simulink model "ImpedanceControl"  (R2017a)
settings: Solver=ode23t  StartTime=0.0  StopTime=10.0  RelTol=1e-1
values from neighbouring files (symbols this model uses):
  Kd = 500*eye(6)    [Initial.m]
  Kp = 2500*eye(6)    [Initial.m]
  Md = 100*eye(6)    [Initial.m]
  Md_inv = inv(Md)    [Initial.m]
libraries: mblibv1 x72
(part 1 of 14)
settings Model: Creator=nathaliemajcherczyk  LastModifiedBy=Nathalie M
settings SolverCC: MaxConsecutiveMinStep=10

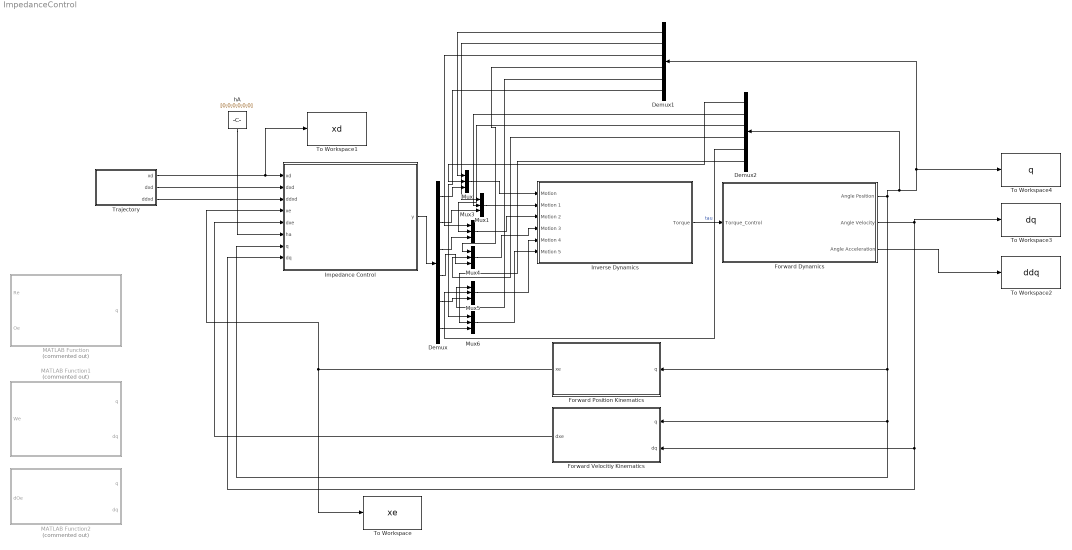
== system ImpedanceControl ==
  Demux : Demux  Outputs=6
  Demux1 : Demux  Outputs=6
  Demux2 : Demux  Outputs=6
  "Forward Dynamics " : Subsystem
  Forward Position Kinematics : MATLAB Function  TreatAsAtomicUnit=on
  Forward Velocitiy Kinematics : MATLAB Function  TreatAsAtomicUnit=on
  Impedance Control : Subsystem
  "Inverse Dynamics " : Subsystem
  MATLAB Function : MATLAB Function  Commented=on  TreatAsAtomicUnit=on
  MATLAB Function1 : MATLAB Function  Commented=on  TreatAsAtomicUnit=on
  MATLAB Function2 : MATLAB Function  Commented=on  TreatAsAtomicUnit=on
  Mux{,1,3..6} (6 alike) : Mux  Inputs=3
  To Workspace : ToWorkspace  VariableName=xe  SaveFormat=Timeseries  SampleTime=-1
  To Workspace1 : ToWorkspace  VariableName=xd  SaveFormat=Timeseries  SampleTime=-1
  To Workspace2 : ToWorkspace  VariableName=ddq  SaveFormat=Timeseries  SampleTime=-1
  To Workspace3 : ToWorkspace  VariableName=dq  SaveFormat=Timeseries  SampleTime=-1
  To Workspace4 : ToWorkspace  VariableName=q  SaveFormat=Timeseries  SampleTime=-1
  Trajectory : Subsystem
  hA : Constant  Value=[0;0;0;0;0;0]
  wires:
  "Forward Dynamics "/1("Angle Position ") -> Demux2/1, To Workspace4/1, Demux1/1, Forward Position Kinematics/1(q), Impedance Control/7(q), Forward Velocitiy Kinematics/1(q)
  "Forward Dynamics "/3(Angle Acceleration) -> To Workspace2/1
  "Forward Dynamics "/2(Angle Velocity) -> To Workspace3/1, Impedance Control/8(dq), Forward Velocitiy Kinematics/2(dq)
  "Inverse Dynamics "/1("Torque ") -> "Forward Dynamics "/1("Torque_Control ")  "tau"
  Impedance Control/1(y) -> Demux/1
  Forward Velocitiy Kinematics/1(dxe) -> Impedance Control/5(dxe)
  Forward Position Kinematics/1(xe) -> Impedance Control/4(xe), To Workspace/1
  hA/1 -> Impedance Control/6(ha)
  Trajectory/1(xd) -> To Workspace1/1, Impedance Control/1(xd)
  Trajectory/2(dxd) -> Impedance Control/2(dxd)
  Trajectory/3(ddxd) -> Impedance Control/3(ddxd)
  Demux/1 -> Mux/3
  Mux/1 -> "Inverse Dynamics "/1("Motion ")
  Demux1/1 -> Mux/1
  Demux2/1 -> Mux/2
  Demux/2 -> Mux1/3
  Mux1/1 -> "Inverse Dynamics "/2(Motion 1)
  Demux1/2 -> Mux1/1
  Demux2/2 -> Mux1/2
  Demux/3 -> Mux3/3
  Demux1/3 -> Mux3/1
  Demux2/3 -> Mux3/2
  Mux3/1 -> "Inverse Dynamics "/3(Motion 2)
  Demux/4 -> Mux4/3
  Mux4/1 -> "Inverse Dynamics "/4(Motion 3)
  Demux1/4 -> Mux4/1
  Demux2/4 -> Mux4/2
  Demux1/6 -> Mux6/1
  Demux/5 -> Mux5/3
  Mux5/1 -> "Inverse Dynamics "/5(Motion 4)
  Demux/6 -> Mux6/3
  Mux6/1 -> "Inverse Dynamics "/6(Motion 5)
  Demux2/6 -> Mux6/2
  Demux1/5 -> Mux5/1
  Demux2/5 -> Mux5/2

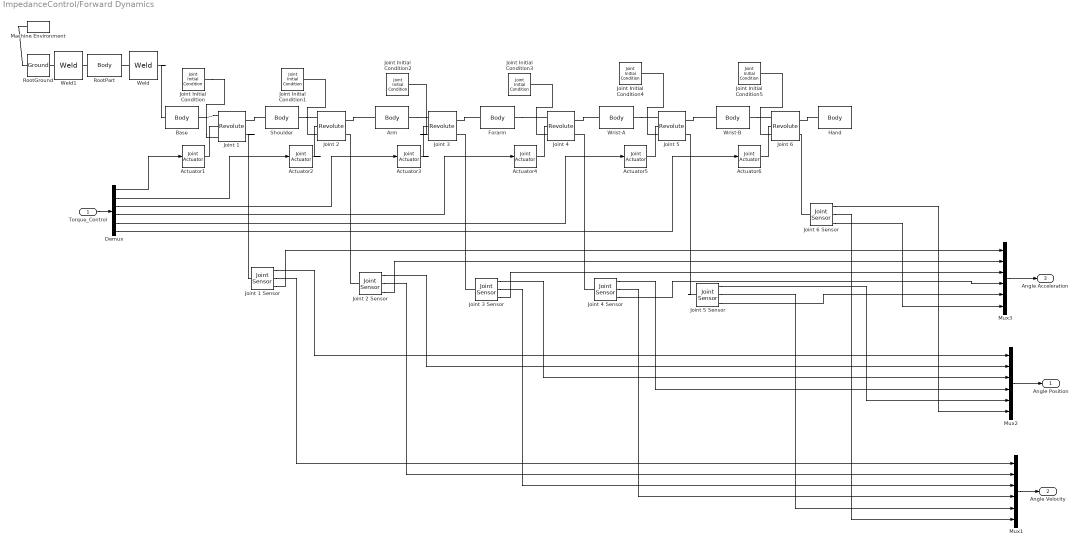
== system ImpedanceControl/Forward Dynamics  ==
  "Torque_Control " : Inport
  Actuator{1..6} (6 alike) : mblibv1/Sensors &  Actuators/Joint Actuator  UpdateFromCAD=off  PhysicalDomain=Mechanical  PortType=blob  ActuationStyle=Force  AngleUnits=deg  ArcVelocityUnits=deg/s  ArcAccelerationUnits=deg/s^2  CoordPositionUnits=m  VelocityUnits=m/s  AccelerationUnits=m/s^2  ForceUnits=N  TorqueUnits=N-m  ActiveIO=on  Width=1  DialogClass=MechanicalActuatorBlock  Primitive=R1  ReferenceFrame=Absolute (World)
      settings: SourceProductName=Simscape Multibody  SourceProductBaseCode=MS
  Arm : mblibv1/Bodies/Body  LConnTagsString=CS2  RConnTagsString=CS3  UpdateFromCAD=on  DialogClass=MechanicalBodyBlock  Mass=1.056  MassUnits=kg  InertiaUnits=kg*m^2  Inertia=[0.0375645,-1.33324e-07,0.000108785;-1.33324e-07,0.0372402,-2.39225e-07;0.000108785,-2.39225e-07,0.00059301]  Shape=Cylinder  ShapeDims=[1 1]  ShapeUnits=m  ShapeUse=false  Density=1  DensityUnits=kg/m^3  DensityUse=false  GraphicsMode=GFXFILE  GraphicsFileName=Jaco_3_7 - arm_ass-1.STL  BodyColorSelMode=COLORPALETTE  BodyColor=[0.752941;0.752941;0.752941]  AttachedToCS=CS1  CG=Right$CG$[0.10282 0.0944444 0.508793]$WORLD$WORLD$m$[0.695251 0.715707 -0.0662524;0.718767 -0.692291 0.0640847;0 -0.092175 -0.995743]$3x3 Transform$rad$WORLD$false$none  WorkingFrames=Right$CS1$[-0.183907 0.105598 0.903425]$WORLD$WORLD$m$[0.695251 0.715707 -0.0662524;0.718767 -0.692291 0.0640847;0 -0.092175 -0.995743]$3x3 Transform$rad$WORLD$false$none#Left$CS2$[0.0767642 0.095252 0.300589]$WORLD$WORLD$m$[1 0 0;0 1 0;0 0 1]$3x3 Transform$rad$WORLD$true$none#Right$CS3$[0.10358 0.0686179 0.708843]$WORLD$WORLD$m$[1 0 0;0 1 0;0 0 1]$3x3 Transform$rad$WORLD$true$none  CGPos=[0.10282 0.0944444 0.508793]  CGRot=[0.695251 0.715707 -0.0662524;0.718767 -0.692291 0.0640847;0 -0.092175 -0.995743]  CS0Pos=[]  CS0Rot=[]  CS1Pos=[-0.183907 0.105598 0.903425]  CS1Rot=[0.695251 0.715707 -0.0662524;0.718767 -0.692291 0.0640847;0 -0.092175 -0.995743]  CS2Pos=[0.0767642 0.095252 0.300589]  CS2Rot=[1 0 0;0 1 0;0 0 1]  CS3Pos=[0.10358 0.0686179 0.708843]  CS3Rot=[1 0 0;0 1 0;0 0 1]  CS4Pos=[]  CS4Rot=[]  CS5Pos=[]  CS5Rot=[]  CS6Pos=[]  CS6Rot=[]  CS7Pos=[]  CS7Rot=[]  CS8Pos=[]  CS8Rot=[]  CS9Pos=[]  CS9Rot=[]  CS10Pos=[]  CS10Rot=[]  CS11Pos=[]  CS11Rot=[]  CS12Pos=[]  CS12Rot=[]  CS13Pos=[]  CS13Rot=[]  CS14Pos=[]  CS14Rot=[]  CS15Pos=[]  CS15Rot=[]  CS16Pos=[]  CS16Rot=[]  CS17Pos=[]  CS17Rot=[]  CS18Pos=[]  CS18Rot=[]  CS19Pos=[]  CS19Rot=[]  CS20Pos=[]  CS20Rot=[]
      settings: SourceProductName=Simscape Multibody  SourceProductBaseCode=MS
  Base : mblibv1/Bodies/Body  LConnTagsString=CS2  RConnTagsString=CS3  UpdateFromCAD=on  DialogClass=MechanicalBodyBlock  Mass=0.570939  MassUnits=kg  InertiaUnits=kg*m^2  Inertia=[0.00175947,1.92772e-07,-3.1782e-05;1.92772e-07,0.00176256,-3.18122e-05;-3.1782e-05,-3.18122e-05,0.000478232]  Shape=Cylinder  ShapeDims=[1 1]  ShapeUnits=m  ShapeUse=false  Density=1  DensityUnits=kg/m^3  DensityUse=false  GraphicsMode=GFXFILE  GraphicsFileName=Jaco_3_7 - base_ass-1.STL  BodyColorSelMode=COLORPALETTE  BodyColor=[0.752941;0.752941;0.752941]  AttachedToCS=CS1  CG=Right$CG$[0.0747134 0.093124 0.128067]$WORLD$WORLD$m$[1 0 0;0 1 0;0 0 1]$3x3 Transform$rad$WORLD$false$none  WorkingFrames=Right$CS1$[0.106448 0.0299726 -0.0762042]$WORLD$WORLD$m$[1 0 0;0 1 0;0 0 1]$3x3 Transform$rad$WORLD$false$none#Left$CS2$[0.0747134 0.093124 0.128067]$WORLD$WORLD$m$[1 0 0;0 1 0;0 0 1]$3x3 Transform$rad$WORLD$true$none#Right$CS3$[0.0753736 0.0938145 0.182089]$WORLD$WORLD$m$[1 0 0;0 1 0;0 0 1]$3x3 Transform$rad$WORLD$true$none  CGPos=[0.0747134 0.093124 0.128067]  CGRot=[1 0 0;0 1 0;0 0 1]  CS0Pos=[]  CS0Rot=[]  CS1Pos=[0.106448 0.0299726 -0.0762042]  CS1Rot=[1 0 0;0 1 0;0 0 1]  CS2Pos=[0.0747134 0.093124 0.128067]  CS2Rot=[1 0 0;0 1 0;0 0 1]  CS3Pos=[0.0753736 0.0938145 0.182089]  CS3Rot=[1 0 0;0 1 0;0 0 1]  CS4Pos=[]  CS4Rot=[]  CS5Pos=[]  CS5Rot=[]  CS6Pos=[]  CS6Rot=[]  CS7Pos=[]  CS7Rot=[]  CS8Pos=[]  CS8Rot=[]  CS9Pos=[]  CS9Rot=[]  CS10Pos=[]  CS10Rot=[]  CS11Pos=[]  CS11Rot=[]  CS12Pos=[]  CS12Rot=[]  CS13Pos=[]  CS13Rot=[]  CS14Pos=[]  CS14Rot=[]  CS15Pos=[]  CS15Rot=[]  CS16Pos=[]  CS16Rot=[]  CS17Pos=[]  CS17Rot=[]  CS18Pos=[]  CS18Rot=[]  CS19Pos=[]  CS19Rot=[]  CS20Pos=[]  CS20Rot=[]
      settings: SourceProductName=Simscape Multibody  SourceProductBaseCode=MS
  Demux : Demux  Outputs=6
  Forarm : mblibv1/Bodies/Body  LConnTagsString=CS2  RConnTagsString=CS3  UpdateFromCAD=on  DialogClass=MechanicalBodyBlock  Mass=0.735414  MassUnits=kg  InertiaUnits=kg*m^2  Inertia=[0.00626271,-0.000115651,1.81814e-08;-0.000115651,0.000377159,4.13244e-07;1.81814e-08,4.13244e-07,0.00610747]  Shape=Cylinder  ShapeDims=[1 1]  ShapeUnits=m  ShapeUse=false  Density=1  DensityUnits=kg/m^3  DensityUse=false  GraphicsMode=GFXFILE  GraphicsFileName=Jaco_3_7 - forarm_ass-1.STL  BodyColorSelMode=COLORPALETTE  BodyColor=[0.752941;0.752941;0.752941]  AttachedToCS=CS1  CG=Right$CG$[0.142291 0.0111153 0.740623]$WORLD$WORLD$m$[0.695251 0.650811 0.305076;0.718767 -0.629518 -0.295094;0 0.424443 -0.905455]$3x3 Transform$rad$WORLD$false$none  WorkingFrames=Right$CS1$[-0.0310579 0.0970807 0.899014]$WORLD$WORLD$m$[0.695251 0.650811 0.305076;0.718767 -0.629518 -0.295094;0 0.424443 -0.905455]$3x3 Transform$rad$WORLD$false$none#Left$CS2$[0.10358 0.0686179 0.708843]$WORLD$WORLD$m$[1 0 0;0 1 0;0 0 1]$3x3 Transform$rad$WORLD$true$none#Right$CS3$[0.230802 -0.0700932 0.796915]$WORLD$WORLD$m$[1 0 0;0 1 0;0 0 1]$3x3 Transform$rad$WORLD$true$none  CGPos=[0.142291 0.0111153 0.740623]  CGRot=[0.695251 0.650811 0.305076;0.718767 -0.629518 -0.295094;0 0.424443 -0.905455]  CS0Pos=[]  CS0Rot=[]  CS1Pos=[-0.0310579 0.0970807 0.899014]  CS1Rot=[0.695251 0.650811 0.305076;0.718767 -0.629518 -0.295094;0 0.424443 -0.905455]  CS2Pos=[0.10358 0.0686179 0.708843]  CS2Rot=[1 0 0;0 1 0;0 0 1]  CS3Pos=[0.230802 -0.0700932 0.796915]  CS3Rot=[1 0 0;0 1 0;0 0 1]  CS4Pos=[]  CS4Rot=[]  CS5Pos=[]  CS5Rot=[]  CS6Pos=[]  CS6Rot=[]  CS7Pos=[]  CS7Rot=[]  CS8Pos=[]  CS8Rot=[]  CS9Pos=[]  CS9Rot=[]  CS10Pos=[]  CS10Rot=[]  CS11Pos=[]  CS11Rot=[]  CS12Pos=[]  CS12Rot=[]  CS13Pos=[]  CS13Rot=[]  CS14Pos=[]  CS14Rot=[]  CS15Pos=[]  CS15Rot=[]  CS16Pos=[]  CS16Rot=[]  CS17Pos=[]  CS17Rot=[]  CS18Pos=[]  CS18Rot=[]  CS19Pos=[]  CS19Rot=[]  CS20Pos=[]  CS20Rot=[]
      settings: SourceProductName=Simscape Multibody  SourceProductBaseCode=MS
  Hand : mblibv1/Bodies/Body  LConnTagsString=CS2  UpdateFromCAD=on  DialogClass=MechanicalBodyBlock  Mass=0.395999  MassUnits=kg  InertiaUnits=kg*m^2  Inertia=[0.00124769,-0.000197969,-5.51354e-06;-0.000197969,0.000409818,-2.12169e-05;-5.51354e-06,-2.12169e-05,0.00139509]  Shape=Cylinder  ShapeDims=[1 1]  ShapeUnits=m  ShapeUse=false  Density=1  DensityUnits=kg/m^3  DensityUse=false  GraphicsMode=GFXFILE  GraphicsFileName=Jaco_3_7 - Hand_ass-1.STL  BodyColorSelMode=COLORPALETTE  BodyColor=[0.752941;0.752941;0.752941]  AttachedToCS=CS1  CG=Right$CG$[0.35442 -0.232757 0.799495]$WORLD$WORLD$m$[-0.439555 0.858973 -0.262597;-0.828489 -0.500657 -0.250895;-0.346983 0.107276 0.931716]$3x3 Transform$rad$WORLD$false$none  WorkingFrames=Right$CS1$[0.362295 -0.115327 0.65151]$WORLD$WORLD$m$[-0.439555 0.858973 -0.262597;-0.828489 -0.500657 -0.250895;-0.346983 0.107276 0.931716]$3x3 Transform$rad$WORLD$false$none#Left$CS2$[0.306767 -0.196631 0.795235]$WORLD$WORLD$m$[1 0 0;0 1 0;0 0 1]$3x3 Transform$rad$WORLD$true$none  CGPos=[0.35442 -0.232757 0.799495]  CGRot=[-0.439555 0.858973 -0.262597;-0.828489 -0.500657 -0.250895;-0.346983 0.107276 0.931716]  CS0Pos=[]  CS0Rot=[]  CS1Pos=[0.362295 -0.115327 0.65151]  CS1Rot=[-0.439555 0.858973 -0.262597;-0.828489 -0.500657 -0.250895;-0.346983 0.107276 0.931716]  CS2Pos=[0.306767 -0.196631 0.795235]  CS2Rot=[1 0 0;0 1 0;0 0 1]  CS3Pos=[]  CS3Rot=[]  CS4Pos=[]  CS4Rot=[]  CS5Pos=[]  CS5Rot=[]  CS6Pos=[]  CS6Rot=[]  CS7Pos=[]  CS7Rot=[]  CS8Pos=[]  CS8Rot=[]  CS9Pos=[]  CS9Rot=[]  CS10Pos=[]  CS10Rot=[]  CS11Pos=[]  CS11Rot=[]  CS12Pos=[]  CS12Rot=[]  CS13Pos=[]  CS13Rot=[]  CS14Pos=[]  CS14Rot=[]  CS15Pos=[]  CS15Rot=[]  CS16Pos=[]  CS16Rot=[]  CS17Pos=[]  CS17Rot=[]  CS18Pos=[]  CS18Rot=[]  CS19Pos=[]  CS19Rot=[]  CS20Pos=[]  CS20Rot=[]
      settings: SourceProductName=Simscape Multibody  SourceProductBaseCode=MS
  Joint 1 : mblibv1/Joints/Revolute  LConnTagsString=__newl0|SA1|SA2  RConnTagsString=__newr0|SA1  UpdateFromCAD=on  NumSAPorts=3  CutJoint=off  MarkAsCut=off  Primitives=prismatic  PrimitiveProps=R1$World$[0,0,1]$revolute  DialogClass=JointBlock  R1Axis=[0,0,1]
      settings: SourceProductName=Simscape Multibody  SourceProductBaseCode=MS
  Joint 1 Sensor : mblibv1/Sensors &  Actuators/Joint Sensor  UpdateFromCAD=off  PhysicalDomain=Mechanical  PortType=blob  Muxed=off  Pose=off  Angle=on  AngleUnits=deg  ArcVelocity=on  ArcVelocityUnits=deg/s  ArcAcceleration=on  ArcAccelerationUnits=deg/s^2  CoordPosition=on  CoordPositionUnits=m  Velocity=off  VelocityUnits=m/s  Acceleration=off  AccelerationUnits=m/s^2  Quaternion=on  QuaternionDT=off  QuaternionDDT=off  QuaternionUnits=off  OutputVector=[1]  ActiveIO=on  Width=3  DialogClass=MechanicalSensorBlock  Primitive=R1  Force=off  ForceUnits=N  Torque=off  TorqueUnits=N*m  ReferenceFrame=Absolute (World)  ReactionSensedSide=Base  ReactionReferenceFrame=Absolute (World)  ReactionForce=off  ReactionForceUnits=N  ReactionMoment=off  ReactionMomentUnits=N*m
      settings: SourceProductName=Simscape Multibody  SourceProductBaseCode=MS
  Joint 2 : mblibv1/Joints/Revolute  LConnTagsString=__newl0|SA1|SA2  RConnTagsString=__newr0|SA1  UpdateFromCAD=on  NumSAPorts=3  CutJoint=off  MarkAsCut=off  Primitives=prismatic  PrimitiveProps=R1$World$[0.695251,0.718767,0]$revolute  DialogClass=JointBlock  R1Axis=[0.695251,0.718767,0]
      settings: SourceProductName=Simscape Multibody  SourceProductBaseCode=MS
  Joint 2 Sensor : mblibv1/Sensors &  Actuators/Joint Sensor  UpdateFromCAD=off  PhysicalDomain=Mechanical  PortType=blob  Muxed=off  Pose=off  Angle=on  AngleUnits=deg  ArcVelocity=on  ArcVelocityUnits=deg/s  ArcAcceleration=on  ArcAccelerationUnits=deg/s^2  CoordPosition=on  CoordPositionUnits=m  Velocity=off  VelocityUnits=m/s  Acceleration=off  AccelerationUnits=m/s^2  Quaternion=on  QuaternionDT=off  QuaternionDDT=off  QuaternionUnits=off  OutputVector=[1]  ActiveIO=on  Width=3  DialogClass=MechanicalSensorBlock  Primitive=R1  Force=off  ForceUnits=N  Torque=off  TorqueUnits=N*m  ReferenceFrame=Absolute (World)  ReactionSensedSide=Base  ReactionReferenceFrame=Absolute (World)  ReactionForce=off  ReactionForceUnits=N  ReactionMoment=off  ReactionMomentUnits=N*m
      settings: SourceProductName=Simscape Multibody  SourceProductBaseCode=MS
  Joint 3 : mblibv1/Joints/Revolute  LConnTagsString=__newl0|SA1|SA2  RConnTagsString=__newr0|SA1  UpdateFromCAD=on  NumSAPorts=3  CutJoint=off  MarkAsCut=off  Primitives=prismatic  PrimitiveProps=R1$World$[-0.695251,-0.718767,0]$revolute  DialogClass=JointBlock  R1Axis=[-0.695251,-0.718767,0]
      settings: SourceProductName=Simscape Multibody  SourceProductBaseCode=MS
  Joint 3 Sensor : mblibv1/Sensors &  Actuators/Joint Sensor  UpdateFromCAD=off  PhysicalDomain=Mechanical  PortType=blob  Muxed=off  Pose=off  Angle=on  AngleUnits=deg  ArcVelocity=on  ArcVelocityUnits=deg/s  ArcAcceleration=on  ArcAccelerationUnits=deg/s^2  CoordPosition=on  CoordPositionUnits=m  Velocity=off  VelocityUnits=m/s  Acceleration=off  AccelerationUnits=m/s^2  Quaternion=on  QuaternionDT=off  QuaternionDDT=off  QuaternionUnits=off  OutputVector=[1]  ActiveIO=on  Width=3  DialogClass=MechanicalSensorBlock  Primitive=R1  Force=off  ForceUnits=N  Torque=off  TorqueUnits=N*m  ReferenceFrame=Absolute (World)  ReactionSensedSide=Base  ReactionReferenceFrame=Absolute (World)  ReactionForce=off  ReactionForceUnits=N  ReactionMoment=off  ReactionMomentUnits=N*m
      settings: SourceProductName=Simscape Multibody  SourceProductBaseCode=MS
  Joint 4 : mblibv1/Joints/Revolute  LConnTagsString=__newl0|SA1|SA2  RConnTagsString=__newr0|SA1  UpdateFromCAD=on  NumSAPorts=3  CutJoint=off  MarkAsCut=off  Primitives=prismatic  PrimitiveProps=R1$World$[0.650811,-0.629518,0.424443]$revolute  DialogClass=JointBlock  R1Axis=[0.650811,-0.629518,0.424443]
      settings: SourceProductName=Simscape Multibody  SourceProductBaseCode=MS
  Joint 4 Sensor : mblibv1/Sensors &  Actuators/Joint Sensor  UpdateFromCAD=off  PhysicalDomain=Mechanical  PortType=blob  Muxed=off  Pose=off  Angle=on  AngleUnits=deg  ArcVelocity=on  ArcVelocityUnits=deg/s  ArcAcceleration=on  ArcAccelerationUnits=deg/s^2  CoordPosition=on  CoordPositionUnits=m  Velocity=off  VelocityUnits=m/s  Acceleration=off  AccelerationUnits=m/s^2  Quaternion=on  QuaternionDT=off  QuaternionDDT=off  QuaternionUnits=off  OutputVector=[1]  ActiveIO=on  Width=3  DialogClass=MechanicalSensorBlock  Primitive=R1  Force=off  ForceUnits=N  Torque=off  TorqueUnits=N*m  ReferenceFrame=Absolute (World)  ReactionSensedSide=Base  ReactionReferenceFrame=Absolute (World)  ReactionForce=off  ReactionForceUnits=N  ReactionMoment=off  ReactionMomentUnits=N*m
      settings: SourceProductName=Simscape Multibody  SourceProductBaseCode=MS
  Joint 5 : mblibv1/Joints/Revolute  LConnTagsString=__newl0|SA1|SA2  RConnTagsString=__newr0|SA1  UpdateFromCAD=on  NumSAPorts=3  CutJoint=off  MarkAsCut=off  Primitives=prismatic  PrimitiveProps=R1$World$[0.15169,-0.946456,-0.284976]$revolute  DialogClass=JointBlock  R1Axis=[0.15169,-0.946456,-0.284976]
      settings: SourceProductName=Simscape Multibody  SourceProductBaseCode=MS
  Joint 5 Sensor : mblibv1/Sensors &  Actuators/Joint Sensor  UpdateFromCAD=off  PhysicalDomain=Mechanical  PortType=blob  Muxed=off  Pose=off  Angle=on  AngleUnits=deg  ArcVelocity=on  ArcVelocityUnits=deg/s  ArcAcceleration=on  ArcAccelerationUnits=deg/s^2  CoordPosition=on  CoordPositionUnits=m  Velocity=off  VelocityUnits=m/s  Acceleration=off  AccelerationUnits=m/s^2  Quaternion=on  QuaternionDT=off  QuaternionDDT=off  QuaternionUnits=off  OutputVector=[1]  ActiveIO=on  Width=3  DialogClass=MechanicalSensorBlock  Primitive=R1  Force=off  ForceUnits=N  Torque=off  TorqueUnits=N*m  ReferenceFrame=Absolute (World)  ReactionSensedSide=Base  ReactionReferenceFrame=Absolute (World)  ReactionForce=off  ReactionForceUnits=N  ReactionMoment=off  ReactionMomentUnits=N*m
      settings: SourceProductName=Simscape Multibody  SourceProductBaseCode=MS
  Joint 6 : mblibv1/Joints/Revolute  LConnTagsString=__newl0|SA1|SA2  RConnTagsString=__newr0|SA1  UpdateFromCAD=on  NumSAPorts=3  CutJoint=off  MarkAsCut=off  Primitives=prismatic  PrimitiveProps=R1$World$[0.858973,-0.500657,0.107276]$revolute  DialogClass=JointBlock  R1Axis=[0.858973,-0.500657,0.107276]
      settings: SourceProductName=Simscape Multibody  SourceProductBaseCode=MS
  Joint 6 Sensor : mblibv1/Sensors &  Actuators/Joint Sensor  UpdateFromCAD=off  PhysicalDomain=Mechanical  PortType=blob  Muxed=off  Pose=off  Angle=on  AngleUnits=deg  ArcVelocity=on  ArcVelocityUnits=deg/s  ArcAcceleration=on  ArcAccelerationUnits=deg/s^2  CoordPosition=on  CoordPositionUnits=m  Velocity=off  VelocityUnits=m/s  Acceleration=off  AccelerationUnits=m/s^2  Quaternion=on  QuaternionDT=off  QuaternionDDT=off  QuaternionUnits=off  OutputVector=[1]  ActiveIO=on  Width=3  DialogClass=MechanicalSensorBlock  Primitive=R1  Force=off  ForceUnits=N  Torque=off  TorqueUnits=N*m  ReferenceFrame=Absolute (World)  ReactionSensedSide=Base  ReactionReferenceFrame=Absolute (World)  ReactionForce=off  ReactionForceUnits=N  ReactionMoment=off  ReactionMomentUnits=N*m
      settings: SourceProductName=Simscape Multibody  SourceProductBaseCode=MS
  Joint Initial Condition : mblibv1/Sensors &  Actuators/Joint Initial Condition  UpdateFromCAD=off  LeftPortType=blob  RightPortType=blob  PhysicalDomain=mechanical  DialogClass=InitialConditionBlock  InitialConditions=P1$false$0$m$deg$0$m/s$deg/s#P2$false$0$m$deg$0$m/s$deg/s#P3$false$0$m$deg$0$m/s$deg/s#R1$true$0.81$m$rad$0$m/s$rad/s#R2$false$0$m$deg$0$m/s$deg/s#R3$false$0$m$deg$0$m/s$deg/s#S$false$0$m$deg$0$m/s$deg/s  P1PIC=0  P1VIC=0  P2PIC=0  P2VIC=0  P3PIC=0  P3VIC=0  R1PIC=0.81  R1VIC=0  R2PIC=0  R2VIC=0  R3PIC=0  R3VIC=0  SPIC=0  SVIC=0
      settings: SourceProductName=Simscape Multibody  SourceProductBaseCode=MS
  Joint Initial Condition1 : mblibv1/Sensors &  Actuators/Joint Initial Condition  UpdateFromCAD=off  LeftPortType=blob  RightPortType=blob  PhysicalDomain=mechanical  DialogClass=InitialConditionBlock  InitialConditions=P1$false$0$m$deg$0$m/s$deg/s#P2$false$0$m$deg$0$m/s$deg/s#P3$false$0$m$deg$0$m/s$deg/s#R1$true$-0.6915$m$rad$0$m/s$rad/s#R2$false$0$m$deg$0$m/s$deg/s#R3$false$0$m$deg$0$m/s$deg/s#S$false$0$m$deg$0$m/s$deg/s  P1PIC=0  P1VIC=0  P2PIC=0  P2VIC=0  P3PIC=0  P3VIC=0  R1PIC=-0.6915  R1VIC=0  R2PIC=0  R2VIC=0  R3PIC=0  R3VIC=0  SPIC=0  SVIC=0
      settings: SourceProductName=Simscape Multibody  SourceProductBaseCode=MS
  Joint Initial Condition2 : mblibv1/Sensors &  Actuators/Joint Initial Condition  UpdateFromCAD=off  LeftPortType=blob  RightPortType=blob  PhysicalDomain=mechanical  DialogClass=InitialConditionBlock  InitialConditions=P1$false$0$m$deg$0$m/s$deg/s#P2$false$0$m$deg$0$m/s$deg/s#P3$false$0$m$deg$0$m/s$deg/s#R1$true$1.5708$m$rad$0.2$m/s$rad/s#R2$false$0$m$deg$0$m/s$deg/s#R3$false$0$m$deg$0$m/s$deg/s#S$false$0$m$deg$0$m/s$deg/s  P1PIC=0  P1VIC=0  P2PIC=0  P2VIC=0  P3PIC=0  P3VIC=0  R1PIC=1.5708  R1VIC=0.2  R2PIC=0  R2VIC=0  R3PIC=0  R3VIC=0  SPIC=0  SVIC=0
      settings: SourceProductName=Simscape Multibody  SourceProductBaseCode=MS
  Joint Initial Condition3 : mblibv1/Sensors &  Actuators/Joint Initial Condition  UpdateFromCAD=off  LeftPortType=blob  RightPortType=blob  PhysicalDomain=mechanical  DialogClass=InitialConditionBlock  InitialConditions=P1$false$0$m$deg$0$m/s$deg/s#P2$false$0$m$deg$0$m/s$deg/s#P3$false$0$m$deg$0$m/s$deg/s#R1$true$3.1415$m$rad$0$m/s$rad/s#R2$false$0$m$deg$0$m/s$deg/s#R3$false$0$m$deg$0$m/s$deg/s#S$false$0$m$deg$0$m/s$deg/s  P1PIC=0  P1VIC=0  P2PIC=0  P2VIC=0  P3PIC=0  P3VIC=0  R1PIC=3.1415  R1VIC=0  R2PIC=0  R2VIC=0  R3PIC=0  R3VIC=0  SPIC=0  SVIC=0
      settings: SourceProductName=Simscape Multibody  SourceProductBaseCode=MS
  Joint Initial Condition4 : mblibv1/Sensors &  Actuators/Joint Initial Condition  UpdateFromCAD=off  LeftPortType=blob  RightPortType=blob  PhysicalDomain=mechanical  DialogClass=InitialConditionBlock  InitialConditions=P1$false$0$m$deg$0$m/s$deg/s#P2$false$0$m$deg$0$m/s$deg/s#P3$false$0$m$deg$0$m/s$deg/s#R1$true$-1.70256$m$rad$0$m/s$deg/s#R2$false$0$m$deg$0$m/s$deg/s#R3$false$0$m$deg$0$m/s$deg/s#S$false$0$m$deg$0$m/s$deg/s  P1PIC=0  P1VIC=0  P2PIC=0  P2VIC=0  P3PIC=0  P3VIC=0  R1PIC=-1.70256  R1VIC=0  R2PIC=0  R2VIC=0  R3PIC=0  R3VIC=0  SPIC=0  SVIC=0
      settings: SourceProductName=Simscape Multibody  SourceProductBaseCode=MS
  Joint Initial Condition5 : mblibv1/Sensors &  Actuators/Joint Initial Condition  UpdateFromCAD=off  LeftPortType=blob  RightPortType=blob  PhysicalDomain=mechanical  DialogClass=InitialConditionBlock  InitialConditions=P1$false$0$m$deg$0$m/s$deg/s#P2$false$0$m$deg$0$m/s$deg/s#P3$false$0$m$deg$0$m/s$deg/s#R1$true$0.8222$m$rad$0$m/s$rad/s#R2$false$0$m$deg$0$m/s$deg/s#R3$false$0$m$deg$0$m/s$deg/s#S$false$0$m$deg$0$m/s$deg/s  P1PIC=0  P1VIC=0  P2PIC=0  P2VIC=0  P3PIC=0  P3VIC=0  R1PIC=0.8222  R1VIC=0  R2PIC=0  R2VIC=0  R3PIC=0  R3VIC=0  SPIC=0  SVIC=0
      settings: SourceProductName=Simscape Multibody  SourceProductBaseCode=MS
  Machine Environment : mblibv1/Bodies/Machine Environment  PortType=env  PhysicalDomain=Mechanical  DialogTemplateClass=MECH.MachineEnvironment  SyncWhenCopied=off  Gravity=[0 0 -9.81]  GravityUnits=m/s^2  GravityAsSignal=off  Dimensionality=Auto-detect  AnalysisType=Forward dynamics  LinearAssemblyTolerance=1e-3  LinearAssemblyToleranceUnits=m  AngularAssemblyTolerance=1e-3  AngularAssemblyToleranceUnits=rad  ConstraintSolverType=Stabilizing  ConstraintRelTolerance=1e-4  ConstraintAbsTolerance=1e-4  UseRobustSingularityHandling=off  RedundancyAnalysisToleranceType=Automatically select tolerance  RedundancyAnalysisTolerance=1e-14  StatePerturbationType=Fixed  PerturbationSize=1e-5  VisualizeMachine=on  BodyVisualizationType=Use model default body geometries  BodyColorSelMode=Use model default  DefaultBodyColor=[1 0 0]
      settings: SourceProductName=Simscape Multibody  SourceProductBaseCode=MS
  Mux1 : Mux  Inputs=6
  Mux2 : Mux  Inputs=6
  Mux3 : Mux  Inputs=6
  RootGround : mblibv1/Bodies/Ground  UpdateFromCAD=on  LeftPortType=env  RightPortType=workingframe  PhysicalDomain=Mechanical  DialogClass=GroundBlock  CoordPosition=[0.154743,0.00421299,0.535333]  CoordPositionUnits=m  StateVectorMgrId=0  MachineId=[1 0]  ShowEnvPort=on  ParameterChecksum=[3417922130, 2383928924, 3577010570, 1911939694]  TopologyChecksum=[2654763649, 4205204799, 1514762018, 2254763851]
      settings: SourceProductName=Simscape Multibody  SourceProductBaseCode=MS
  RootPart : mblibv1/Bodies/Body  LConnTagsString=CS3  RConnTagsString=CS2  UpdateFromCAD=on  DialogClass=MechanicalBodyBlock  Mass=0  MassUnits=kg  InertiaUnits=kg*m^2  Inertia=[0,0,0;0,0,0;0,0,0]  Shape=Cylinder  ShapeDims=[1 1]  ShapeUnits=m  ShapeUse=false  Density=1  DensityUnits=kg/m^3  DensityUse=false  GraphicsMode=MACHINE_DEFAULT  BodyColorSelMode=MACHINE_DEFAULT  BodyColor=[1;0;0]  AttachedToCS=CS1  CG=Right$CG$[0.154743 0.00421299 0.535333]$WORLD$WORLD$m$[1 0 0;0 1 0;0 0 1]$3x3 Transform$rad$WORLD$false$none  WorkingFrames=Right$CS1$[0 0 0]$WORLD$WORLD$m$[1 0 0;0 1 0;0 0 1]$3x3 Transform$rad$WORLD$false$none#Right$CS2$[0.0747134 0.093124 0.128067]$WORLD$WORLD$m$[1 0 0;0 1 0;0 0 1]$3x3 Transform$rad$WORLD$true$none#Left$CS3$[0.154743 0.00421299 0.535333]$WORLD$WORLD$m$[1 0 0;0 1 0;0 0 1]$3x3 Transform$rad$WORLD$true$none  CGPos=[0.154743 0.00421299 0.535333]  CGRot=[1 0 0;0 1 0;0 0 1]  CS0Pos=[]  CS0Rot=[]  CS1Pos=[0 0 0]  CS1Rot=[1 0 0;0 1 0;0 0 1]  CS2Pos=[0.0747134 0.093124 0.128067]  CS2Rot=[1 0 0;0 1 0;0 0 1]  CS3Pos=[0.154743 0.00421299 0.535333]  CS3Rot=[1 0 0;0 1 0;0 0 1]  CS4Pos=[]  CS4Rot=[]  CS5Pos=[]  CS5Rot=[]  CS6Pos=[]  CS6Rot=[]  CS7Pos=[]  CS7Rot=[]  CS8Pos=[]  CS8Rot=[]  CS9Pos=[]  CS9Rot=[]  CS10Pos=[]  CS10Rot=[]  CS11Pos=[]  CS11Rot=[]  CS12Pos=[]  CS12Rot=[]  CS13Pos=[]  CS13Rot=[]  CS14Pos=[]  CS14Rot=[]  CS15Pos=[]  CS15Rot=[]  CS16Pos=[]  CS16Rot=[]  CS17Pos=[]  CS17Rot=[]  CS18Pos=[]  CS18Rot=[]  CS19Pos=[]  CS19Rot=[]  CS20Pos=[]  CS20Rot=[]
      settings: SourceProductName=Simscape Multibody  SourceProductBaseCode=MS
  Shoulder : mblibv1/Bodies/Body  LConnTagsString=CS3  RConnTagsString=CS2  UpdateFromCAD=on  DialogClass=MechanicalBodyBlock  Mass=0.813994  MassUnits=kg  InertiaUnits=kg*m^2  Inertia=[0.0026546,0.000304923,5.38935e-08;0.000304923,0.000595598,-3.17242e-07;5.38935e-08,-3.17242e-07,0.00258406]  Shape=Cylinder  ShapeDims=[1 1]  ShapeUnits=m  ShapeUse=false  Density=1  DensityUnits=kg/m^3  DensityUse=false  GraphicsMode=GFXFILE  GraphicsFileName=Jaco_3_7 - shoulder_ass-1.STL  BodyColorSelMode=COLORPALETTE  BodyColor=[0.752941;0.752941;0.752941]  AttachedToCS=CS1  CG=Right$CG$[0.0698164 0.0880634 0.250193]$WORLD$WORLD$m$[0.695251 0 0.718767;0.718767 0 -0.695251;0 1 0]$3x3 Transform$rad$WORLD$false$none  WorkingFrames=Right$CS1$[-0.0564522 0.142463 0.184725]$WORLD$WORLD$m$[0.695251 0 0.718767;0.718767 0 -0.695251;0 1 0]$3x3 Transform$rad$WORLD$false$none#Right$CS2$[0.0767642 0.095252 0.300589]$WORLD$WORLD$m$[1 0 0;0 1 0;0 0 1]$3x3 Transform$rad$WORLD$true$none#Left$CS3$[0.0753736 0.0938145 0.182089]$WORLD$WORLD$m$[1 0 0;0 1 0;0 0 1]$3x3 Transform$rad$WORLD$true$none  CGPos=[0.0698164 0.0880634 0.250193]  CGRot=[0.695251 0 0.718767;0.718767 0 -0.695251;0 1 0]  CS0Pos=[]  CS0Rot=[]  CS1Pos=[-0.0564522 0.142463 0.184725]  CS1Rot=[0.695251 0 0.718767;0.718767 0 -0.695251;0 1 0]  CS2Pos=[0.0767642 0.095252 0.300589]  CS2Rot=[1 0 0;0 1 0;0 0 1]  CS3Pos=[0.0753736 0.0938145 0.182089]  CS3Rot=[1 0 0;0 1 0;0 0 1]  CS4Pos=[]  CS4Rot=[]  CS5Pos=[]  CS5Rot=[]  CS6Pos=[]  CS6Rot=[]  CS7Pos=[]  CS7Rot=[]  CS8Pos=[]  CS8Rot=[]  CS9Pos=[]  CS9Rot=[]  CS10Pos=[]  CS10Rot=[]  CS11Pos=[]  CS11Rot=[]  CS12Pos=[]  CS12Rot=[]  CS13Pos=[]  CS13Rot=[]  CS14Pos=[]  CS14Rot=[]  CS15Pos=[]  CS15Rot=[]  CS16Pos=[]  CS16Rot=[]  CS17Pos=[]  CS17Rot=[]  CS18Pos=[]  CS18Rot=[]  CS19Pos=[]  CS19Rot=[]  CS20Pos=[]  CS20Rot=[]
      settings: SourceProductName=Simscape Multibody  SourceProductBaseCode=MS
  Weld : mblibv1/Joints/Weld  LConnTagsString=__newl0  RConnTagsString=__newr0  UpdateFromCAD=on  NumSAPorts=0  CutJoint=off  MarkAsCut=off  Primitives=weld  PrimitiveProps=W$WORLD$[0.57735,0.57735,0.57735]$weld  DialogClass=JointBlock  WAxis=[0.57735,0.57735,0.57735]
      settings: SourceProductName=Simscape Multibody  SourceProductBaseCode=MS
  Weld1 : mblibv1/Joints/Weld  LConnTagsString=__newl0  RConnTagsString=__newr0  UpdateFromCAD=on  NumSAPorts=0  CutJoint=off  MarkAsCut=off  Primitives=weld  PrimitiveProps=W$WORLD$[0.57735,0.57735,0.57735]$weld  DialogClass=JointBlock  WAxis=[0.57735,0.57735,0.57735]
      settings: SourceProductName=Simscape Multibody  SourceProductBaseCode=MS
  Wrist-A : mblibv1/Bodies/Body  LConnTagsString=CS3  RConnTagsString=CS2  UpdateFromCAD=on  DialogClass=MechanicalBodyBlock  Mass=0.44698  MassUnits=kg  InertiaUnits=kg*m^2  Inertia=[0.000407036,-3.06246e-08,5.0605e-09;-3.06246e-08,0.000239744,-8.7175e-05;5.0605e-09,-8.7175e-05,0.000376656]  Shape=Cylinder  ShapeDims=[1 1]  ShapeUnits=m  ShapeUse=false  Density=1  DensityUnits=kg/m^3  DensityUse=false  GraphicsMode=GFXFILE  GraphicsFileName=Jaco_3_7 - wrist1_ass-1.STL  BodyColorSelMode=COLORPALETTE  BodyColor=[0.752941;0.752941;0.752941]  AttachedToCS=CS1  CG=Right$CG$[0.251866 -0.101707 0.805258]$WORLD$WORLD$m$[0.709409 0.650811 -0.270524;0.30501 -0.629518 -0.714616;-0.63538 0.424443 -0.64509]$3x3 Transform$rad$WORLD$false$none  WorkingFrames=Right$CS1$[0.228148 -0.0304193 0.852839]$WORLD$WORLD$m$[0.709409 0.650811 -0.270524;0.30501 -0.629518 -0.714616;-0.63538 0.424443 -0.64509]$3x3 Transform$rad$WORLD$false$none#Right$CS2$[0.264276 -0.136155 0.802577]$WORLD$WORLD$m$[1 0 0;0 1 0;0 0 1]$3x3 Transform$rad$WORLD$true$none#Left$CS3$[0.230802 -0.0700932 0.796915]$WORLD$WORLD$m$[1 0 0;0 1 0;0 0 1]$3x3 Transform$rad$WORLD$true$none  CGPos=[0.251866 -0.101707 0.805258]  CGRot=[0.709409 0.650811 -0.270524;0.30501 -0.629518 -0.714616;-0.63538 0.424443 -0.64509]  CS0Pos=[]  CS0Rot=[]  CS1Pos=[0.228148 -0.0304193 0.852839]  CS1Rot=[0.709409 0.650811 -0.270524;0.30501 -0.629518 -0.714616;-0.63538 0.424443 -0.64509]  CS2Pos=[0.264276 -0.136155 0.802577]  CS2Rot=[1 0 0;0 1 0;0 0 1]  CS3Pos=[0.230802 -0.0700932 0.796915]  CS3Rot=[1 0 0;0 1 0;0 0 1]  CS4Pos=[]  CS4Rot=[]  CS5Pos=[]  CS5Rot=[]  CS6Pos=[]  CS6Rot=[]  CS7Pos=[]  CS7Rot=[]  CS8Pos=[]  CS8Rot=[]  CS9Pos=[]  CS9Rot=[]  CS10Pos=[]  CS10Rot=[]  CS11Pos=[]  CS11Rot=[]  CS12Pos=[]  CS12Rot=[]  CS13Pos=[]  CS13Rot=[]  CS14Pos=[]  CS14Rot=[]  CS15Pos=[]  CS15Rot=[]  CS16Pos=[]  CS16Rot=[]  CS17Pos=[]  CS17Rot=[]  CS18Pos=[]  CS18Rot=[]  CS19Pos=[]  CS19Rot=[]  CS20Pos=[]  CS20Rot=[]
      settings: SourceProductName=Simscape Multibody  SourceProductBaseCode=MS
  Wrist-B : mblibv1/Bodies/Body  LConnTagsString=CS3  RConnTagsString=CS2  UpdateFromCAD=on  DialogClass=MechanicalBodyBlock  Mass=0.44698  MassUnits=kg  InertiaUnits=kg*m^2  Inertia=[0.000407036,-3.06246e-08,5.0605e-09;-3.06246e-08,0.000239744,-8.7175e-05;5.0605e-09,-8.7175e-05,0.000376656]  Shape=Cylinder  ShapeDims=[1 1]  ShapeUnits=m  ShapeUse=false  Density=1  DensityUnits=kg/m^3  DensityUse=false  GraphicsMode=GFXFILE  GraphicsFileName=Jaco_3_7 - wrist2_ass-1.STL  BodyColorSelMode=COLORPALETTE  BodyColor=[0.752941;0.752941;0.752941]  AttachedToCS=CS1  CG=Right$CG$[0.28076 -0.170724 0.795794]$WORLD$WORLD$m$[-0.298122 0.15169 0.942398;-0.318695 -0.946456 0.0515257;0.899754 -0.284976 0.330502]$3x3 Transform$rad$WORLD$false$none  WorkingFrames=Right$CS1$[0.211333 -0.128563 0.759589]$WORLD$WORLD$m$[-0.298122 0.15169 0.942398;-0.318695 -0.946456 0.0515257;0.899754 -0.284976 0.330502]$3x3 Transform$rad$WORLD$false$none#Right$CS2$[0.306767 -0.196631 0.795235]$WORLD$WORLD$m$[1 0 0;0 1 0;0 0 1]$3x3 Transform$rad$WORLD$true$none#Left$CS3$[0.264276 -0.136155 0.802577]$WORLD$WORLD$m$[1 0 0;0 1 0;0 0 1]$3x3 Transform$rad$WORLD$true$none  CGPos=[0.28076 -0.170724 0.795794]  CGRot=[-0.298122 0.15169 0.942398;-0.318695 -0.946456 0.0515257;0.899754 -0.284976 0.330502]  CS0Pos=[]  CS0Rot=[]  CS1Pos=[0.211333 -0.128563 0.759589]  CS1Rot=[-0.298122 0.15169 0.942398;-0.318695 -0.946456 0.0515257;0.899754 -0.284976 0.330502]  CS2Pos=[0.306767 -0.196631 0.795235]  CS2Rot=[1 0 0;0 1 0;0 0 1]  CS3Pos=[0.264276 -0.136155 0.802577]  CS3Rot=[1 0 0;0 1 0;0 0 1]  CS4Pos=[]  CS4Rot=[]  CS5Pos=[]  CS5Rot=[]  CS6Pos=[]  CS6Rot=[]  CS7Pos=[]  CS7Rot=[]  CS8Pos=[]  CS8Rot=[]  CS9Pos=[]  CS9Rot=[]  CS10Pos=[]  CS10Rot=[]  CS11Pos=[]  CS11Rot=[]  CS12Pos=[]  CS12Rot=[]  CS13Pos=[]  CS13Rot=[]  CS14Pos=[]  CS14Rot=[]  CS15Pos=[]  CS15Rot=[]  CS16Pos=[]  CS16Rot=[]  CS17Pos=[]  CS17Rot=[]  CS18Pos=[]  CS18Rot=[]  CS19Pos=[]  CS19Rot=[]  CS20Pos=[]  CS20Rot=[]
      settings: SourceProductName=Simscape Multibody  SourceProductBaseCode=MS
  "Angle Position " : Outport
  Angle Velocity : Outport  Port=2
  Angle Acceleration : Outport  Port=3
  wires:
  Demux/2 -> Actuator2/1
  Demux/3 -> Actuator3/1
  Demux/4 -> Actuator4/1
  Demux/5 -> Actuator5/1
  Demux/6 -> Actuator6/1
  Joint 3 Sensor/1 -> Mux2/3
  Joint 6 Sensor/1 -> Mux2/6
  Joint 6 Sensor/2 -> Mux1/6
  Demux/1 -> Actuator1/1
  "Torque_Control "/1 -> Demux/1
  Mux2/1 -> "Angle Position "/1
  Joint 1 Sensor/1 -> Mux2/1
  Joint 2 Sensor/1 -> Mux2/2
  Joint 4 Sensor/1 -> Mux2/4
  Joint 5 Sensor/1 -> Mux2/5
  Mux1/1 -> Angle Velocity/1
  Joint 1 Sensor/2 -> Mux1/1
  Joint 2 Sensor/2 -> Mux1/2
  Joint 3 Sensor/2 -> Mux1/3
  Joint 4 Sensor/2 -> Mux1/4
  Joint 5 Sensor/2 -> Mux1/5
  Mux3/1 -> Angle Acceleration/1
  Joint 6 Sensor/3 -> Mux3/6
  Joint 5 Sensor/3 -> Mux3/5
  Joint 4 Sensor/3 -> Mux3/4
  Joint 3 Sensor/3 -> Mux3/3
  Joint 2 Sensor/3 -> Mux3/2
  Joint 1 Sensor/3 -> Mux3/1
  connections:
  Actuator5/RConn1 -- Joint 5/LConn2
  Shoulder/RConn1 -- Joint 2/LConn1
  Joint 3 Sensor/LConn1 -- Joint 3/RConn2
  Weld/RConn1 -- Base/LConn1
  Joint 3/RConn1 -- Forarm/LConn1
  Joint 5/RConn1 -- Wrist-B/LConn1
  Joint 6/RConn1 -- Hand/LConn1
  Joint 6 Sensor/LConn1 -- Joint 6/RConn2
  Joint 2/RConn1 -- Arm/LConn1
  Actuator3/RConn1 -- Joint 3/LConn2
  Joint 5 Sensor/LConn1 -- Joint 5/RConn2
  Joint 4 Sensor/LConn1 -- Joint 4/RConn2
  Arm/RConn1 -- Joint 3/LConn1
  Actuator6/RConn1 -- Joint 6/LConn2
  Actuator4/RConn1 -- Joint 4/LConn2
  Joint 1/RConn1 -- Shoulder/LConn1
  RootPart/RConn1 -- Weld/LConn1
  Base/RConn1 -- Joint 1/LConn1
  Wrist-A/RConn1 -- Joint 5/LConn1
  Wrist-B/RConn1 -- Joint 6/LConn1
  Weld1/RConn1 -- RootPart/LConn1
  Joint 4/RConn1 -- Wrist-A/LConn1
  Forarm/RConn1 -- Joint 4/LConn1
  Joint 2 Sensor/LConn1 -- Joint 2/RConn2
  RootGround/RConn1 -- Weld1/LConn1
  Actuator2/RConn1 -- Joint 2/LConn2
  Joint 1/LConn2 -- Actuator1/RConn1
  Joint 1/RConn2 -- Joint 1 Sensor/LConn1
  Machine Environment/RConn1 -- RootGround/LConn1
  Joint 2/LConn3 -- Joint Initial Condition1/RConn1
  Joint 5/LConn3 -- Joint Initial Condition4/RConn1
  Joint 4/LConn3 -- Joint Initial Condition3/RConn1
  Joint 3/LConn3 -- Joint Initial Condition2/RConn1
  Joint 6/LConn3 -- Joint Initial Condition5/RConn1
  Joint Initial Condition/RConn1 -- Joint 1/LConn3

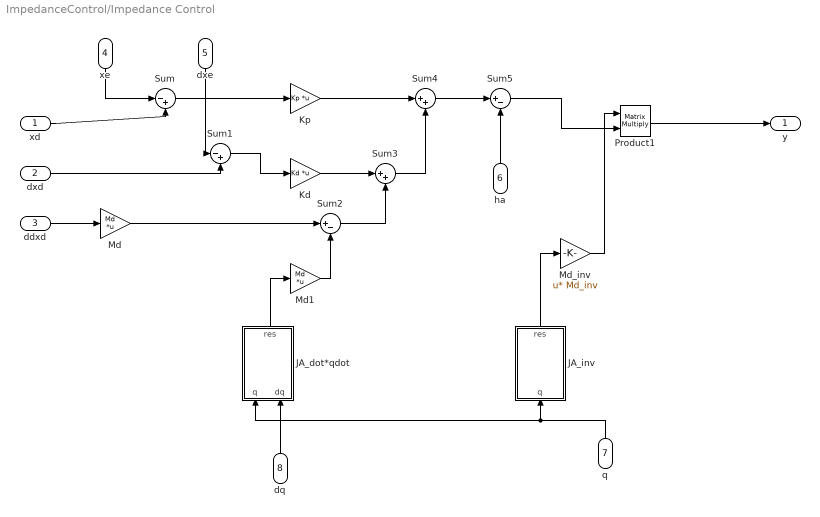
== system ImpedanceControl/Impedance Control ==
  xd : Inport
  dxd : Inport  Port=2
  ddxd : Inport  Port=3
  xe : Inport  Port=4
  dxe : Inport  Port=5
  ha : Inport  Port=6
  q : Inport  Port=7
  dq : Inport  Port=8
  JA_dot*qdot : MATLAB Function  TreatAsAtomicUnit=on
  JA_inv : MATLAB Function  TreatAsAtomicUnit=on
  Kd : Gain  Gain=Kd  Multiplication=Matrix(K*u)
  Kp : Gain  Gain=Kp  Multiplication=Matrix(K*u)
  Md : Gain  Gain=Md  Multiplication=Matrix(K*u)
  Md1 : Gain  Gain=Md  Multiplication=Matrix(K*u)
  Md_inv : Gain  Gain=Md_inv  Multiplication=Matrix(u*K)
  Product1 : Product  Multiplication=Matrix(*)
  Sum : Sum  Inputs=|-+
  Sum1 : Sum  Inputs=|-+
  Sum2 : Sum  Inputs=|+-
  Sum3 : Sum  Inputs=|++
  Sum4 : Sum  Inputs=|++
  Sum5 : Sum  Inputs=|+-
  y : Outport
  wires:
  xd/1 -> Sum/2
  dxd/1 -> Sum1/2
  ddxd/1 -> Md/1
  xe/1 -> Sum/1
  Sum/1 -> Kp/1
  dxe/1 -> Sum1/1
  Sum1/1 -> Kd/1
  JA_inv/1(res) -> Md_inv/1
  q/1 -> JA_dot*qdot/1(q), JA_inv/1(q)
  Md_inv/1 -> Product1/1
  dq/1 -> JA_dot*qdot/2(dq)
  JA_dot*qdot/1(res) -> Md1/1
  Md1/1 -> Sum2/2
  Md/1 -> Sum2/1
  Sum2/1 -> Sum3/2
  Kd/1 -> Sum3/1
  Sum3/1 -> Sum4/2
  Kp/1 -> Sum4/1
  ha/1 -> Sum5/2
  Sum4/1 -> Sum5/1
  Sum5/1 -> Product1/2
  Product1/1 -> y/1
